simulink subsystem "ComputeL"  (R2020b)
settings: Solver=VariableStepAuto  StartTime=0.0  StopTime=10.0  RelTol=1e-3
settings Model: Creator=marco  LastModifiedBy=marco

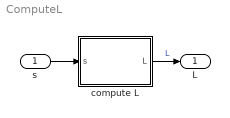
== system ComputeL ==
  s : Inport
  compute L : MATLAB Function  TreatAsAtomicUnit=on
  L : Outport
  wires:
  compute L/1(L) -> L/1  "L"
  s/1 -> compute L/1(s)

== matlab function ComputeL/compute L ==
  data: s input; L output
function L = fcn(s)

L = computeL(s);
